simulink model "FlyingSheet_simulator"  (R2019b)
settings: Solver=VariableStepAuto  StartTime=0.0  StopTime=30  RelTol=1e-3
values from neighbouring files (symbols this model uses):
  p =     [ds.mat]    (also in vxs.mat)
undefined symbols (not defined in the file or in its folder): quatnormalize
libraries: aerolibutil x24, simulink x14, sharedtransform x6, vrlib x4, sharedutil x3, simulink_extras x2, dspsrcs4 x1, aerolibanim x1, aerolibanimutils x1
(part 2 of 2)

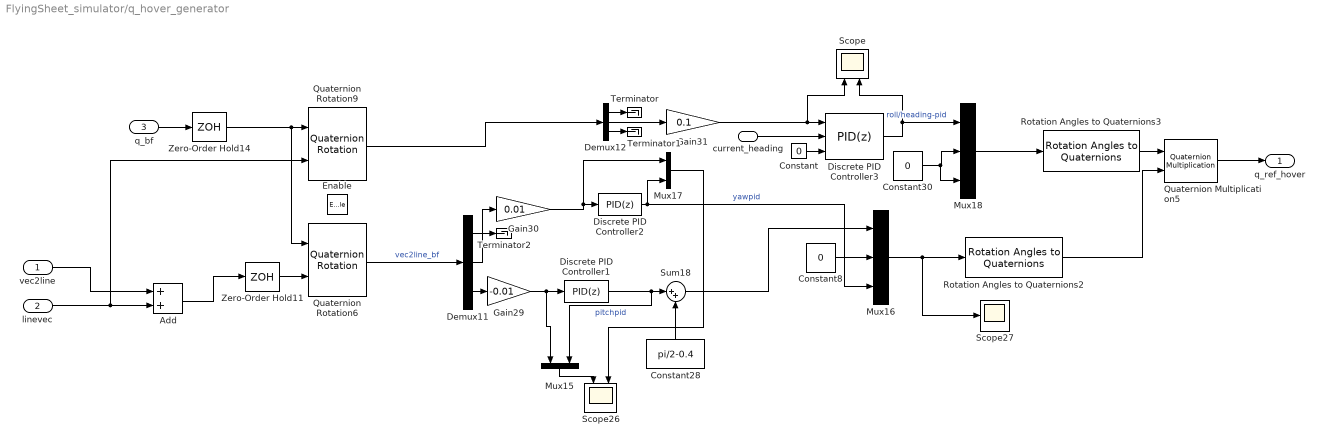
== system FlyingSheet_simulator/q_hover_generator ==
  vec2line : Inport
  linevec : Inport  Port=2
  q_bf : Inport  Port=3
  current_heading : Inport  Port=4
  Enable : EnablePort  StatesWhenEnabling=reset
  Add : Sum
  Constant : Constant  Value=0
  Constant28 : Constant  Value=pi/2-0.4
  Constant30 : Constant  Value=0
  Constant8 : Constant  Value=0
  Demux11 : Demux  Outputs=3
  Demux12 : Demux  Outputs=3
  Discrete PID Controller1 : simulink/Continuous/PID Controller  Controller=PID  Form=Parallel  TimeDomain=Discrete-time  SampleTime=-1  IntegratorMethod=Forward Euler  FilterMethod=Forward Euler  ControllerParametersSource=internal  P=0.75  I=0.1  D=8  UseFilter=off  N=100  TunerSelectOption=Transfer Function Based (PID Tuner App)  InitialConditionSource=internal  InitialConditionForIntegrator=0  InitialConditionForFilter=0  DifferentiatorICPrevScaledInput=0  ExternalReset=none  TrackingMode=off  Kt=1  LimitOutput=on  UpperSaturationLimit=deg2rad(40)  LowerSaturationLimit=-deg2rad(40)  LinearizeAsGain=off  AntiWindupMode=none  Kb=1  POutMin=[]  POutMax=[]  IOutMin=[]  IOutMax=[]  DOutMin=[]  DOutMax=[]  NOutMin=[]  NOutMax=[]  SumOutMin=[]  SumOutMax=[]  SaturationOutMin=[]  SaturationOutMax=[]  PParamMin=[]  PParamMax=[]  IParamMin=[]  IParamMax=[]  DParamMin=[]  DParamMax=[]  NParamMin=[]  NParamMax=[]  KbParamMin=[]  KbParamMax=[]  KtParamMin=[]  KtParamMax=[]  KbOutMin=[]  KbOutMax=[]  KtOutMin=[]  KtOutMax=[]  IntegratorOutMin=[]  IntegratorOutMax=[]  FilterOutMin=[]  FilterOutMax=[]  SumI1OutMin=[]  SumI1OutMax=[]  SumI2OutMin=[]  SumI2OutMax=[]  SumI3OutMin=[]  SumI3OutMax=[]  SumI4OutMin=[]  SumI4OutMax=[]  SumDOutMin=[]  SumDOutMax=[]  DifferentiatorOutMin=[]  DifferentiatorOutMax=[]  FilterDiffOutCoefMin=[]  FilterDiffOutCoefMax=[]  ReciprocalOutMin=[]  ReciprocalOutMax=[]  SumDenOutMin=[]  SumDenOutMax=[]  SumNumOutMin=[]  SumNumOutMax=[]  DivideOutMin=[]  DivideOutMax=[]  IntegratorContinuousStateAttributes=''  IntegratorStateMustResolveToSignalObject=off  IntegratorRTWStateStorageClass=Auto  FilterContinuousStateAttributes=''  FilterStateMustResolveToSignalObject=off  FilterRTWStateStorageClass=Auto  ParallelPVariant=InternalParameters  IdealPVariant=Disabled  IVariant=InternalParameters  DVariant=InternalParameters  IntegratorVariant=Discrete  SatVariant=Enabled  AWVariant=Passthrough  PCopyVariant=Disabled  TRVariant=Disabled  FdbkBlocksVariant=Forward  IdealPFdbkVariant=Disabled  SatFdbkVariant=Disabled  DerivativeFilterVariant=Differentiator  NVariant=Passthrough  NCopyVariant=Disabled_SignalSpec  FilterICVariant=InternalICsDifferentiator  IntegratorICVariant=InternalICs  ExternalResetVariant=Disabled  TRSumVariant=Passthrough  SumFdbkVariant=Disabled  SumVariant=Sum_PID
  Discrete PID Controller2 : simulink/Continuous/PID Controller  Controller=PID  Form=Parallel  TimeDomain=Discrete-time  SampleTime=-1  IntegratorMethod=Forward Euler  FilterMethod=Forward Euler  ControllerParametersSource=internal  P=1  I=0  D=2  UseFilter=off  N=100  TunerSelectOption=Transfer Function Based (PID Tuner App)  InitialConditionSource=internal  InitialConditionForIntegrator=0  InitialConditionForFilter=0  DifferentiatorICPrevScaledInput=0  ExternalReset=none  TrackingMode=off  Kt=1  LimitOutput=on  UpperSaturationLimit=deg2rad(40)  LowerSaturationLimit=-deg2rad(40)  LinearizeAsGain=off  AntiWindupMode=none  Kb=1  POutMin=[]  POutMax=[]  IOutMin=[]  IOutMax=[]  DOutMin=[]  DOutMax=[]  NOutMin=[]  NOutMax=[]  SumOutMin=[]  SumOutMax=[]  SaturationOutMin=[]  SaturationOutMax=[]  PParamMin=[]  PParamMax=[]  IParamMin=[]  IParamMax=[]  DParamMin=[]  DParamMax=[]  NParamMin=[]  NParamMax=[]  KbParamMin=[]  KbParamMax=[]  KtParamMin=[]  KtParamMax=[]  KbOutMin=[]  KbOutMax=[]  KtOutMin=[]  KtOutMax=[]  IntegratorOutMin=[]  IntegratorOutMax=[]  FilterOutMin=[]  FilterOutMax=[]  SumI1OutMin=[]  SumI1OutMax=[]  SumI2OutMin=[]  SumI2OutMax=[]  SumI3OutMin=[]  SumI3OutMax=[]  SumI4OutMin=[]  SumI4OutMax=[]  SumDOutMin=[]  SumDOutMax=[]  DifferentiatorOutMin=[]  DifferentiatorOutMax=[]  FilterDiffOutCoefMin=[]  FilterDiffOutCoefMax=[]  ReciprocalOutMin=[]  ReciprocalOutMax=[]  SumDenOutMin=[]  SumDenOutMax=[]  SumNumOutMin=[]  SumNumOutMax=[]  DivideOutMin=[]  DivideOutMax=[]  IntegratorContinuousStateAttributes=''  IntegratorStateMustResolveToSignalObject=off  IntegratorRTWStateStorageClass=Auto  FilterContinuousStateAttributes=''  FilterStateMustResolveToSignalObject=off  FilterRTWStateStorageClass=Auto  ParallelPVariant=InternalParameters  IdealPVariant=Disabled  IVariant=InternalParameters  DVariant=InternalParameters  IntegratorVariant=Discrete  SatVariant=Enabled  AWVariant=Passthrough  PCopyVariant=Disabled  TRVariant=Disabled  FdbkBlocksVariant=Forward  IdealPFdbkVariant=Disabled  SatFdbkVariant=Disabled  DerivativeFilterVariant=Differentiator  NVariant=Passthrough  NCopyVariant=Disabled_SignalSpec  FilterICVariant=InternalICsDifferentiator  IntegratorICVariant=InternalICs  ExternalResetVariant=Disabled  TRSumVariant=Passthrough  SumFdbkVariant=Disabled  SumVariant=Sum_PID
  Discrete PID Controller3 : simulink/Continuous/PID Controller  Controller=PID  Form=Parallel  TimeDomain=Discrete-time  SampleTime=-1  IntegratorMethod=Forward Euler  FilterMethod=Forward Euler  ControllerParametersSource=internal  P=1  I=1  D=0  UseFilter=off  N=100  TunerSelectOption=Transfer Function Based (PID Tuner App)  InitialConditionSource=external  InitialConditionForIntegrator=0  InitialConditionForFilter=0  DifferentiatorICPrevScaledInput=0  ExternalReset=none  TrackingMode=off  Kt=1  LimitOutput=off  UpperSaturationLimit=deg2rad(40)  LowerSaturationLimit=-deg2rad(40)  LinearizeAsGain=off  AntiWindupMode=none  Kb=1  POutMin=[]  POutMax=[]  IOutMin=[]  IOutMax=[]  DOutMin=[]  DOutMax=[]  NOutMin=[]  NOutMax=[]  SumOutMin=[]  SumOutMax=[]  SaturationOutMin=[]  SaturationOutMax=[]  PParamMin=[]  PParamMax=[]  IParamMin=[]  IParamMax=[]  DParamMin=[]  DParamMax=[]  NParamMin=[]  NParamMax=[]  KbParamMin=[]  KbParamMax=[]  KtParamMin=[]  KtParamMax=[]  KbOutMin=[]  KbOutMax=[]  KtOutMin=[]  KtOutMax=[]  IntegratorOutMin=[]  IntegratorOutMax=[]  FilterOutMin=[]  FilterOutMax=[]  SumI1OutMin=[]  SumI1OutMax=[]  SumI2OutMin=[]  SumI2OutMax=[]  SumI3OutMin=[]  SumI3OutMax=[]  SumI4OutMin=[]  SumI4OutMax=[]  SumDOutMin=[]  SumDOutMax=[]  DifferentiatorOutMin=[]  DifferentiatorOutMax=[]  FilterDiffOutCoefMin=[]  FilterDiffOutCoefMax=[]  ReciprocalOutMin=[]  ReciprocalOutMax=[]  SumDenOutMin=[]  SumDenOutMax=[]  SumNumOutMin=[]  SumNumOutMax=[]  DivideOutMin=[]  DivideOutMax=[]  IntegratorContinuousStateAttributes=''  IntegratorStateMustResolveToSignalObject=off  IntegratorRTWStateStorageClass=Auto  FilterContinuousStateAttributes=''  FilterStateMustResolveToSignalObject=off  FilterRTWStateStorageClass=Auto  ParallelPVariant=InternalParameters  IdealPVariant=Disabled  IVariant=InternalParameters  DVariant=InternalParameters  IntegratorVariant=Discrete  SatVariant=Disabled  AWVariant=Passthrough  PCopyVariant=Disabled  TRVariant=Disabled  FdbkBlocksVariant=Forward  IdealPFdbkVariant=Disabled  SatFdbkVariant=Disabled  DerivativeFilterVariant=Differentiator  NVariant=Passthrough  NCopyVariant=Disabled_SignalSpec  FilterICVariant=ExternalICs  IntegratorICVariant=ExternalICs  ExternalResetVariant=Disabled  TRSumVariant=Passthrough  SumFdbkVariant=Disabled  SumVariant=Sum_PID
  Gain29 : Gain  Gain=-0.01
  Gain30 : Gain  Gain=0.01
  Gain31 : Gain  Gain=0.1
  Mux15 : Mux  Inputs=2
  Mux16 : Mux  Inputs=3
  Mux17 : Mux  Inputs=2
  Mux18 : Mux  Inputs=3
  Quaternion Multiplication5 : aerolibutil/Quaternion Multiplication
  Quaternion Rotation6 : aerolibutil/Quaternion Rotation
  Quaternion Rotation9 : aerolibutil/Quaternion Rotation
  Rotation Angles to Quaternions2 : sharedtransform/Rotation Angles to Quaternions  rotationOrder=YXZ  aMode=aMode
      settings: SourceProductName=Aerospace Blockset  SourceProductBaseCode=AE
  Rotation Angles to Quaternions3 : sharedtransform/Rotation Angles to Quaternions  rotationOrder=ZYX  aMode=aMode
      settings: SourceProductName=Aerospace Blockset  SourceProductBaseCode=AE
  Scope : Scope  NumInputPorts=2
  Scope26 : Scope  NumInputPorts=2
  Scope27 : Scope
  Sum18 : Sum  Inputs=|++
  Terminator : Terminator
  Terminator1 : Terminator
  Terminator2 : Terminator
  Zero-Order Hold11 : ZeroOrderHold  SampleTime=p.Ts
  Zero-Order Hold14 : ZeroOrderHold  SampleTime=p.Ts
  q_ref_hover : Outport  VectorParamsAs1DForOutWhenUnconnected=off
  wires:
  vec2line/1 -> Add/1
  Discrete PID Controller1/1 -> Sum18/1, Mux15/2  "pitchpid"
  Gain29/1 -> Mux15/1, Discrete PID Controller1/1
  Demux11/2 -> Gain30/1
  Quaternion Rotation6/1 -> Demux11/1  "vec2line_bf"
  Constant30/1 -> Mux18/3, Mux18/2
  Demux12/3 -> Terminator1/1
  Demux12/1 -> Terminator/1
  Gain31/1 -> Scope/1, Discrete PID Controller3/1
  linevec/1 -> Quaternion Rotation9/2, Add/2
  Discrete PID Controller3/1 -> Scope/2, Mux18/1  "roll/heading-pid"
  Mux15/1 -> Scope26/1
  Mux16/1 -> Scope27/1, Rotation Angles to Quaternions2/1
  Rotation Angles to Quaternions3/1 -> Quaternion Multiplication5/1
  q_bf/1 -> Zero-Order Hold14/1
  Demux11/3 -> Gain29/1
  Constant8/1 -> Mux16/2
  Discrete PID Controller2/1 -> Mux16/3, Mux17/2  "yawpid"
  Rotation Angles to Quaternions2/1 -> Quaternion Multiplication5/2
  Mux18/1 -> Rotation Angles to Quaternions3/1
  Quaternion Multiplication5/1 -> q_ref_hover/1
  Demux12/2 -> Gain31/1
  Mux17/1 -> Scope26/2
  Add/1 -> Zero-Order Hold11/1
  Zero-Order Hold14/1 -> Quaternion Rotation6/1, Quaternion Rotation9/1
  Constant28/1 -> Sum18/2
  Gain30/1 -> Mux17/1, Discrete PID Controller2/1
  Zero-Order Hold11/1 -> Quaternion Rotation6/2
  Demux11/1 -> Terminator2/1
  Sum18/1 -> Mux16/1
  Constant/1 -> Discrete PID Controller3/3
  current_heading/1 -> Discrete PID Controller3/2
  Quaternion Rotation9/1 -> Demux12/1

== matlab function FlyingSheet_simulator/Torque_FL ==
  data: u_omegaL output; u_omegaR output; u_deltaL output; u_deltaR output; tao input; states input; u_jointT input; p parameter
function [u_omegaL,u_omegaR, u_deltaL,u_deltaR]  = FL_torques(tao, states, u_jointT, p)


wxr = tao(1); % I wonder if this comversion from omega to tao is right? Depends on Emil Fresk implementation
wyr = tao(2);
wzr = tao(3);
v = states(1:3);
vx = v(1);
vy = v(2);
vz = v(3);
w = states(4:6);
wx = w(1);
wy = w(2);
wz = w(3);
q = states(7:10); % Possibly not needed?
q0=q(1);
q1=q(2);
q2=q(3);
q3=(4);
deltaL = states(11);
deltaR = states(12);
omegaL = states(13);
omegaR = states(14);

% init output vector
u_deltaL = 0;
u_deltaR = 0;
u_omegaL = 0;
u_omegaR = 0;

% If you know of a better way (not counting modifying the code below to use
% p.x notation, plese feel welcome to tell me.
%P = struct2cell(p);
%Pn = fieldnames(p);
%for i=1:numel(P)
%    eval(Pn{i}+"="+string(P{i})+";")
%end
Ts=p.Ts;
m=p.m;
Ix=p.Ix;
Iy=p.Iy;
Iz=p.Iz;
I=p.I;
g=p.g;
rho=p.rho;
propd=p.propd;
K_T=p.K_T;
K_v=p.K_v;
b_w=p.b_w;
Sa=p.Sa;
Saw=p.Saw;
CLdelta=p.CLdelta;
CDdelta=p.CDdelta;
SW=p.SW;
Sw_w=p.Sw_w;
Sw=p.Sw;
b=p.b;
Cmyl=p.Cmyl;
Cwy=p.Cwy;
yf=p.yf;
yt=p.yt;
xW=p.xW;
xf=p.xf;
xac=p.xac;
zW=p.zW;
yw=p.yw;
yW=p.yW;
yWE=p.yWE;
yWEE=p.yWEE;
K_omegaL=p.K_omegaL;
K_omegaR=p.K_omegaR;
K_deltaL=p.K_deltaL;
K_deltaR=p.K_deltaR;
CL_A=p.CL_A;
CL_B=p.CL_B;
CL_C=p.CL_C;
CD_A=p.CD_A;
CD_B=p.CD_B;
CD_C=p.CD_C;
CLB_A=p.CLB_A;
CLB_B=p.CLB_B;
CDB_A=p.CDB_A;
CDB_B=p.CDB_B;
% The constants below are for the polynomial approximations.
% I am lookin into a way of auto-generating them in a struct or something.
a11=p.a11;
a12=p.a12;
a13=p.a13;
a21=p.a21;
a22=p.a22;
a23=p.a23;
a31=p.a31;
a32=p.a32;
a33=p.a33;
a41=p.a41;
a42=p.a42;
a43=p.a43;
b11=p.b11;
b12=p.b12;
b13=p.b13;
b14=p.b14;
b21=p.b21;
b22=p.b22;
b23=p.b23;
b24=p.b24;
b31=p.b31;
b32=p.b32;
b33=p.b33;
b34=p.b34;
c11=p.c11;
c12=p.c12;
c13=p.c13;
c14=p.c14;
c21=p.c21;
c22=p.c22;
c23=p.c23;
c24=p.c24;
c31=p.c31;
c32=p.c32;
c33=p.c33;
c34=p.c34;
c41=p.c41;
c42=p.c42;
c43=p.c43;
c44=p.c44;
% Assuming we made correct choices here it should suffice with this:
%u = [u_deltaA u_jointA u_deltaT]';


% Hey, anyone reading this? Code below is auto-generated because the
% F.L. was just too much of a headache to do
% manyally, so I wrote a script for it.
wn = p.wn;
u_ref =[ ...
];
 
u_deltaA = u_ref(1);
u_jointA = u_ref(2);
u_deltaT = u_ref(3);

u_deltaL = u_jointA - u_deltaA/2;
u_deltaR = u_jointA + u_deltaA/2;
u_omegaL = u_jointT + u_deltaT/2;
u_omegaR = u_jointT - u_deltaT/2;

gain = 1;
u_deltaL = gain*u_deltaL;
u_deltaR = gain*u_deltaR;

end

== matlab function FlyingSheet_simulator/TailSitter/tailsittersimv2 ==
  data: omegaLdot output; omegaRdot output; deltaLdot output; deltaRdot output; qdot output; wdot output; vdot output; omegaL input; omegaR input; deltaL input; deltaR input; u_omegaL input; u_omegaR input; u_deltaL input; u_deltaR input; q input; w input; v input; wind_v input; p parameter; alpha output; Beta output; g_out output
function [ omegaLdot, omegaRdot, deltaLdot, deltaRdot, qdot,wdot,vdot, alpha, Beta, g_out] = ...
    tailsitter_v2(omegaL, omegaR, deltaL, deltaR, u_omegaL, u_omegaR, u_deltaL, ...
    u_deltaR, q,w,v, wind_v, p)

% Set output port dim
omegaLdot = 0;
omegaRdot = 0;
deltaLdot = 0;
deltaRdot = 0;
alpha = 0;
Beta = 0;
qdot = zeros(4,1);
wdot = zeros(3,1);
vdot = zeros(3,1);
g_out = zeros(3,1);

% Map inputs
vx = v(1) + wind_v(1);
vy = v(2) + wind_v(2);
vz = v(3) + wind_v(3);

wx = w(1);
wy = w(2);
wz = w(3);

q0 = q(1);
q1 = q(2);
q2 = q(3);
q3 = q(4);

% function handles not supported, so adding here directly
c = @(y) 0.39; % This should be pretty accurate
% Lift curves
CL = @(alpha) p.CL_A*sin(p.CL_B.*alpha)+p.CL_C; % These are wrong, just placeholders
CD = @(alpha) p.CD_A-p.CD_A.*cos(p.CD_B.*alpha)+p.CD_C;

alpha = atan2(vz,vx);

%Thrust
TL = p.K_T .* omegaL.^2;
TR = p.K_T .* omegaR.^2;

% airflow in thrust wake
v_w_L = p.b_w .* omegaL; %[b_w .* omegaL; vy; vz];
v_w_R = p.b_w .* omegaR;
%alpha_wL = atan2(vz,v_w_L);
%alpha_wR = atan2(vz,v_w_R);

% Quaternion
qdot = 0.5.*[-q1 -q2 -q3; ...
            q0 -q3 q2; ...
            q3 q0 -q1; ...
            -q2 q1 q0]*w;

% inputs
deltaLdot = p.K_deltaL .* (-deltaL + u_deltaL);
deltaRdot = p.K_deltaR .* (-deltaR + u_deltaR);
omegaLdot = p.K_omegaL .* (-omegaL + u_omegaL);
omegaRdot = p.K_omegaR .* (-omegaR + u_omegaR);

% gravity
% To get vector g in bf from wf
% we need to rotate it by q_wf, or conj(q_bf)
qc = quatconj([q0 q1 q2 q3]); %
qc0 = qc(1);
qc1 = qc(2);
qc2 = qc(3);
qc3 = qc(4);
gravity = p.g .* [2.*(qc1.*qc3 + qc0.*qc2); ...
                2.*(qc2.*qc3 - qc0.*qc1); ...
                (qc0.^2 - qc1.^2 - qc2.^2 + qc3.^2);
                zeros(3+4+4,1)];
g_out = gravity(1:3,1);
% Inertial forces
inertialF = -[2*(vz.*wy - vy.*wz); ...
             2*(vx.*wz - vz.*wx); ...
             2*(vy.*wx - vx.*wy); ...
             (p.Iz - p.Iy).*wy.*wz./p.Ix; ...
             (p.Ix - p.Iz).*wx.*wz./p.Iy; ...
             (p.Iy - p.Ix).*wx.*wy./p.Iz; ...
             zeros(8,1)];
%Sideslip
Beta = atan2(vy,vx);

% Winglets
CLB = @(beta) p.CLB_A*sin(p.CLB_B.*beta); % These are wrong, just placeholders
CDB = @(beta) p.CDB_A-p.CDB_A.*cos(p.CDB_B.*beta);
L_W = -p.rho * sqrt(vx.^2+vy.^2) * p.SW * (CLB(Beta)*vx + CDB(Beta)*vy); % Lift in bodyframe, y
D_W = p.rho * sqrt(vx.^2+vy.^2) * p.SW * (-CLB(Beta)*vy + CDB(Beta)*vx); % Drag in bodyfram, x

% MAIN WING
% Lift inside wake
LLT = p.Sw_w * 0.5 * p.rho * abs(v_w_L) .* CL(0).*v_w_L ;
LRT = p.Sw_w * 0.5 * p.rho * abs(v_w_R) .* CL(0).*v_w_R ;
% Lift outside wake
LL = p.Sw * 0.5 * p.rho * sqrt(vx.^2 + vz.^2) .* ...
    (CL(alpha).*vx + CD(alpha).*vz);
LR = LL; % Yeah we -could- combine these, but too late!
% Drag inside wake
DLT = p.Sw_w * 0.5 * p.rho * abs(v_w_L) * CD(0) * v_w_L;
DRT = p.Sw_w * 0.5 * p.rho * abs(v_w_R) * CD(0) * v_w_R;
% Drag outside wake
DL = p.Sw * 0.5 * p.rho * sqrt(vx.^2  + vz.^2) .* ...
    (-CL(alpha).*vz + CD(alpha).*vx);
DR = DL; % Yeah, we -could- combine these as well...

% AILERONS
% Lift inside wake, signs bc rotation dir of aileron
FLT = -p.CLdelta * 0.5*p.rho*v_w_L.^2 * p.Saw * deltaL;
FRT = -p.CLdelta * 0.5*p.rho*v_w_R.^2 * p.Saw * deltaR;
% Lift outside wake
FL = -sign(vx).*p.CLdelta * 0.5*p.rho*(vx.^2 + vy.^2 + vz.^2) * p.Sa * deltaL;
FR = -sign(vx).*p.CLdelta * 0.5*p.rho*(vx.^2 + vy.^2 + vz.^2) * p.Sa * deltaR;
% Drag inside wake
DalphaLT =p.CDdelta * 0.5*p.rho*v_w_L.^2 * p.Saw * abs(deltaL);
DalphaRT = p.CDdelta * 0.5*p.rho*v_w_R.^2 * p.Saw * abs(deltaR);
% Drag outside wake, we add sign of vx because we might be reversing?
DalphaL = sign(vx).*p.CDdelta * 0.5*p.rho*(vx.^2 + vy.^2 + vz.^2) * p.Sa * abs(deltaL);
DalphaR = sign(vx).*p.CDdelta * 0.5*p.rho*(vx.^2 + vy.^2 + vz.^2) * p.Sa * abs(deltaR);

% f1
 % diff in ail deflection
  % inside wake
  % outside wake
 % resmom roll,
 % roll due to yaw rate
 % moment due to sideslip
alphal_rmr = @(y) atan2(vz+wx.*y, vx);
restmomroll = @(y) y .* c(y) .* sqrt(vx.^2 + (vz+wx.*y).^2) .* ...
    (CL(alphal_rmr(y)).*vx + CD(alphal_rmr(y)).*(vz+wx.*y));
alphal_rwz = @(y) atan2(vz, vx-wz.*y);
rollduetowz = @(y) y .* c(y) .* sqrt((vx-wz.*y).^2 + vz.^2) .* ...
    (CL(alphal_rwz(y)).*(vx-wz*y) + CD(alphal_rwz(y)).*vz);
f1 = p.yf.*(FLT+FL -FRT-FR) ...
    -0.5*p.rho.*quadgk(restmomroll,-p.yW,p.yW) ... % between wakes
     -0.5*p.rho.*quadgk(restmomroll,-p.yWEE,-p.yWE) ... % outside left wake
      -0.5*p.rho.*quadgk(restmomroll,p.yWE,p.yWEE) ... % outside right wake
    -0.5*p.rho.*quadgk(rollduetowz,-p.yW,p.yW) ... between wakes
     -0.5*p.rho.*quadgk(rollduetowz,-p.yWEE,-p.yWE) ... left side
      -0.5*p.rho.*quadgk(rollduetowz, p.yWE,p.yWEE) ... right side
    +p.zW*L_W;
% f2
 % joint ail deflection
  % inside wake
  % outside wake
 % pitch moment
 % restmom pitch rate, --- compensate for wake!
 % Pitch from winglets
f2 = p.xf.*(FLT+FL+FRT+FR) ...
    ... %+ 0.5*p.rho*p.Cmyl*(2*p.Sw.*(vx.^2+vy.^2+vz.^2)+p.Sw_w*(v_w_L.^2 + v_w_R.^2) ) ...
    -p.xac.*(LL+LR+LLT+LRT) ... % We do not assume Pith coeff static.
    -wy.*p.rho.*2.*p.Sw.*p.Cwy.*sqrt(vx.^2 + vz.^2) ...
    +p.zW*D_W;
% f3
 % diff in T
 % mom due to sideslip
 % restmom yaw rate, compensate for outside wake
restmomwz = @(y) y .* c(y) .* sqrt((vx-wz.*y).^2 + vz.^2) .* ...
    (-CL(alphal_rwz(y)).*vz + CD(alphal_rwz(y)).*(vx-wz.*y));
f3 = p.yt.*(TL-TR) ...
     -p.xW*L_W ...
     +0.5*quadgk(restmomwz,-p.yW,p.yW) ...
     +0.5*quadgk(restmomwz,-p.yWEE,-p.yWE) ...
     +0.5*quadgk(restmomwz, p.yWE,p.yWEE);
 
%velocities
vxdot = (TL +TR -DL -DR -DLT -DRT -D_W -DalphaL -DalphaR -DalphaLT -DalphaRT)./p.m;
vydot = L_W./p.m;
vzdot = (-LL -LR -LLT -LRT +FL +FR +FLT +FRT)./p.m;

% angular rates
wxdot = f1./p.Ix;
wydot = f2./p.Iy;
wzdot = f3./p.Iz;

%if any(abs(vxdot) > 100)
%    p.m
%end

statesdot = gravity + inertialF +  ...
    [vxdot;vydot;vzdot;wxdot;wydot;wzdot;qdot;...
    deltaLdot;deltaRdot;omegaLdot;omegaRdot];

vdot = statesdot(1:3);
wdot = statesdot(4:6);
qdot = statesdot(7:10);
deltaLdot = statesdot(11);
deltaRdot = statesdot(12);
omegaLdot = statesdot(13);
omegaRdot = statesdot(14);

== matlab function FlyingSheet_simulator/TailSitter/myQuatNorm ==
  data: q input; n output
function n = fcn(q)

n = sqrt(q(1).^2 + q(2).^2 + q(3).^2 + q(4).^2);

== matlab function FlyingSheet_simulator/MATLAB Function ==
  data: u input; y output
function y = norm(u)

y = sqrt(sum(u.^2));

== matlab function FlyingSheet_simulator/TailSitter/MATLAB Function ==
  data: time input; w output
function w = rotsteps(time)

stept = 10;
wt = 10;
reverse = 0;
if time<stept
    w = [0.1,0,0];
elseif time<stept+wt
    if reverse
        w = [-0.1,0,0];
    else
        w = zeros(1,3);
    end
elseif time<2*stept+wt
    w = [0,0,0.1];
elseif time<2*stept+2*wt
    if reverse
        w = [0,0,-0.1];
    else
        w = zeros(1,3);
    end
else
    w = [0,0.1,0];
end

== matlab function FlyingSheet_simulator/MATLAB Function2 ==
  data: q_wf input; q_ref output
function q_ref = refquat(q_wf)

% TODO: Figure out how to set a good reference quaternion.
q_ref = q_wf;

== matlab function FlyingSheet_simulator/MATLAB Function1 ==
  data: v_ref input; q_ref output; u_jointT output
function [q_ref,u_jointT] = ref_quat(v_ref)


q_ref = [1,0,0,0]';
u_jointT = 300;

% We have output of 5dof.
% Input is 3dof.
% We can extend input dof by saying we want wings to be horizontal, now
% total in is 4dof.


%Construct quaterion from several different rotations?

== matlab function FlyingSheet_simulator/linegenerator ==
  settings: updateMethod=DISCRETE
  data: v_wf input; r input; p parameter; rspeed output; wpN output; dist2wp output; linevec output; vec2line output; wp_r output
function [rspeed,wpN, dist2wp, linevec, vec2line, wp_r] = LineGenerator( v_wf,r, p)

% Keep track of which waypoint we are going to
persistent waypointno;
persistent wp;
persistent wp_prev;
persistent miss;
if isempty(waypointno)
    waypointno=2;
    wp=p.waypoints(waypointno,:)';
    wp_prev=p.waypoints(waypointno-1,:)';
    miss=0;
end

%initialize variables
dist2line2d = 0;
altError = 0;
thetaerr = 0;
rspeed = 0;
vec2line = [0,0,0]';

% if current waypoint is the start wp/home wp jump immediately to next.
dist2wp = sqrt( sum( (wp(1:3)-r).^2 ) );
if dist2wp <= wp(5)
    if waypointno < p.numwp
        waypointno = waypointno+1;
    else
        waypointno = 2; % we always skip home wp at origin
    end
    wp_prev = wp;
    wp = p.waypoints(waypointno,:)';
    miss=0;
end
rspeed = wp(4);
wp_r = wp(1:3); % Next waypoint position, v has been scaled away thus wp_r

% find vector between last waypoint and current target
linevec = (wp(1:3)-wp_prev(1:3))./sqrt( sum((wp(1:3)-wp_prev(1:3)).^2) );

% Check if we missed our goal!
%{
if ~miss && dot(linevec, wp(1:3)-r) < 0 && sqrt(sum( (wp(1:3)-r).^2 )) > wp(5)*2
    linevec(1:2)=-linevec(1:2);
    miss=1;
elseif miss
    linevec(1:2)=-linevec(1:2);
end
%}
if  dot(linevec, wp(1:3)-r) < 0 
    linevec(1:3)=-linevec(1:3);
end
% Figure out if goal is ahead of us or if we passed it/missed it.
%if dot(v_wf(1:3), wp(1:3)-r(1:3)) < 0
%    linevec(1:2) = - linevec(1:2);
%end
% THe above doesn't work.

%{
% find angle in x-y plane of vector
thetastar = atan2(linevec(2), linevec(1));
% find our current heading
theta = atan2(v_wf(2),v_wf(1));
% Error in direction along line / be paralell with line
thetaerr = thetastar - theta;
%}

% Find the vector that describes the vector to the closest point on the
% line
a = wp_prev(1:3);               % Points to "start of line"
n = linevec;                    % Points toward next wp
vec2line = a-r - dot(a-r,n)*n;
%altError = vec2line(3);
%dist2line2d = sqrt( sum( vec2line(1:2).^2 ));
wpN = waypointno;


% Mix the vectors for reference according to how far away from line we are

% Old setup, constants: 0.0075/0.01, max/dl2coeff
%{
%cr = cross(linevec,vec2line);
%refvec = linevec;
vcomp = (12/rspeed).^2;
if abs(d2lcoeff*dist2line2d) < max2l*vcomp
    refvec = linevec + d2lcoeff*dist2line2d*vec2line;
else
    refvec = linevec + vcomp*max2l*vec2line;
end
}
%}

%{
vcomp=1/rspeed;
refvec = linevec+vec2line*d2lcoeff*vcomp;

refvec = refvec/sqrt(sum(refvec.^2));
%}

== matlab function FlyingSheet_simulator/q_fly_generator/MATLAB Function3 ==
  data: pitchPID input; vherror output; pitch output; vr_wf input; v_wf input
function [vherror,pitch] = setpitch(pitchPID,vr_wf, v_wf)

pitch = 0;

% Angle toward horizon given by:
horzspeedr = sqrt(sum(vr_wf(1:2).^2));  % Horizontal speed requested
pitch = (horzspeedr +6.013)/15.38;      % From simulations and linefitting
pitch = (pi/2-pitch);                   % correct for coordsys

% We can choose:
%   - Regulate horizontal speed with pitch and altitude with engine power
%   - Regulate horizontal speed with engine power and altitude with pitch.
%
% The first option makes sense when hovering but may be problematic when
% flying: if we are horizontally oriented and dropping in altitude engine
% power cannot do anything about it. However, it will try to increase speed
% forcing the pitch controller to pitch up to reduce speed. Might work.
% The second option makes sense when flying. When hovering we have no
% horizontal speed though.
%

horzspeed  = sqrt(sum( v_wf(1:2).^2));  % Actual horizontal speed
vherror = horzspeedr-horzspeed;         % Error in horizontal speed, to be
                                        % sent to externa PID.

% correct pitch using measurments, use external pid
pitch = pitch + pitchPID;


% use error in direction to roll slightly, use external PID
%roll = 0.1*yawe;

== matlab function FlyingSheet_simulator/MATLAB Function9 ==
  data: q_fly input; vr_wf input; v_cutoff input; q_ref output; q_hover input; hovermode output
function [q_ref, hovermode] = modeswitcher(q_fly, vr_wf, v_cutoff, q_hover)

hspeed = sqrt(sum( vr_wf(1:2).^2 ));
vspeed = abs(vr_wf(3));

Theta = atan2(hspeed, vspeed);

rspeed = sqrt(sum( vr_wf.^2 ));
if rspeed < v_cutoff || abs(Theta) < deg2rad(20)
    q_ref = q_hover;
    hovermode = 1;
else
    q_ref = q_fly;
    hovermode=0;
end

== matlab function FlyingSheet_simulator/linegenerator1 ==
  settings: updateMethod=DISCRETE
  data: max2l input; d2lcoeff input; r input; altError output; p parameter; rspeed output; refvec output; wpN output; dist2wp output; vec2line output
function [altError, rspeed, refvec, wpN, dist2wp, vec2line] = LineGenerator(max2l, d2lcoeff ,r,p)

% Keep track of which waypoint we are going to
persistent waypointno;
persistent wp;
persistent wp_prev;
if isempty(waypointno)
    waypointno = 1;
    wp = p.waypoints(waypointno,:)';
    wp_prev = p.waypoints(waypointno,:)';
end

%initialize variables
dist2line2d = 0;
altError = 0;
rspeed = 0;
vec2line = [0,0,0]';

% if current waypoint is the start wp/home wp jump immediately to next.
dist2wp = sqrt( sum( (wp(1:3)-r).^2 ) );
if dist2wp <= p.wpradius
    if waypointno < p.numwp
        waypointno = waypointno+1;
    else
        waypointno = 1; 
    end
    wp_prev = wp;
    wp = p.waypoints(waypointno,:)';
end
rspeed = wp(4);

% find vector between last waypoint and current target
linevec = (wp(1:3)-wp_prev(1:3))./sqrt( sum((wp(1:3)-wp_prev(1:3)).^2) );

% Figure out if goal is ahead of us or if we passed it/missed it.
%if dot(v_wf(1:3), wp(1:3)-r(1:3)) < 0
%    linevec(1:2) = - linevec(1:2);
%end
% THe above doesn't work.


% Find the vector that describes the vector to the closest point on the
% line
a = wp_prev(1:3);
n = linevec;
vec2line = a-r - dot(a-r,n)*n;
altError = vec2line(3);
dist2line2d = sqrt( sum( vec2line(1:2).^2 ));
wpN = waypointno;


% Mix the vectors for reference according to how far away from line we are
%cr = cross(linevec,vec2line);
%refvec = linevec;
if abs(d2lcoeff*dist2line2d) < max2l
    refvec = linevec + d2lcoeff*dist2line2d*vec2line;
else
    refvec = linevec + max2l*vec2line;
end
refvec = refvec/sqrt(sum(refvec.^2));

== matlab function FlyingSheet_simulator/q_fly_generator/ZYX-quat ==
  data: y input; z input; q output; x input
function q = rotang2quat(y,z,x)

q = [0,0,0,0];

u = [z,y,x];
qa = quaternion(u, 'euler', 'ZYX', 'frame');
q = qa.compact;

== matlab function FlyingSheet_simulator/q_fly_generator/MATLAB Function5 ==
  data: yawr input; yaw input; yawe output
function yawe = fcn(yawr,yaw)

% IF our angle error is more than 180 degrees we need to cross the sign
% barrier, this code should take care of that.
% Since rate limiters are in play, we might need to loo at yawr_target, but
% lets wait with that for now.

yawe = yawr-yaw;
% r:100, y:-90 => e=190 => -360+190= -170
% r:-100, y=90 => e=-190 => 360+(-190) = 170
if yawe > pi
    yawe = -2*pi+yawe;
elseif yawe < -pi
    yawe = 2*pi+yawe;
end

== matlab function FlyingSheet_simulator/q_fly_generator/MATLAB Function6 ==
  data: yawr input; maxrate input; yawr_last input; yawr_slow output; p parameter
function yawr_slow  = fcn(yawr, maxrate, yawr_last, p)

%This is a rate limiter that takes into account which direction is closest
%to the reference, i.e. makes sure we cross the sign at +-pi if we need to.

% We would like to set yawr_slow to yawr, but can only approach it in steps
% of maxrate.
yawr_slow = yawr;
e = yawr-yawr_last;
% slew rate = unit/s => (unit*sampletime)/s
maxrate = maxrate*p.Ts;

if abs(e) > maxrate
    if e > pi
        yawr_slow = yawr_last - maxrate;
    elseif e < -pi
        yawr_slow = yawr_last + maxrate;
    else
        yawr_slow = yawr_last + sign(e)*maxrate;
    end
end

while(yawr_slow > pi)
    yawr_slow = yawr_slow - 2*pi;
end
while(yawr_slow < -pi)
    yawr_slow = yawr_slow + 2*pi;
end

end

== matlab function FlyingSheet_simulator/MATLAB Function7 ==
  data: refvec input; qref output
function qref = refvec2refquat(refvec)

qref = [0,0,0,0];

% set yaw correct
if sqrt(sum( refvec(1:2).^2 )) < 0.1 % Check if we are only pointing up
    Y = 0;
else
    Y = atan2(refvec(2),refvec(1));
end
qY = [cos(Y/2),0,0,sin(Y/2)];

% set pitch correct
hspeed = sqrt(sum(refvec(1:2)).^2);
T = atan2(refvec(3),hspeed);
qT = [cos(T/2),0,sin(T/2),0];


% Set roll to horizontal
qR = [1,0,0,0];

qref = quatmultiply(quatmultiply(qY,qT), qR);

== matlab function FlyingSheet_simulator/q_fly_generator/MATLAB Function8 ==
  data: vr_wf input; yawr output; v_wf input; yaw output
function [yawr,yaw] = setyaw(vr_wf,v_wf)

% reference heading
yawr = atan2(vr_wf(2),vr_wf(1));
%current heading
 yaw = atan2(v_wf(2),v_wf(1));

== matlab function FlyingSheet_simulator/FlyVecAdjust ==
  data: rspeed input; refvec output; vec2line input; linevec input; d2lcoeff input
function refvec = flyVecAdjust(rspeed, vec2line,linevec, d2lcoeff)

vcomp=1/rspeed;
refvec = linevec+vec2line*d2lcoeff*vcomp;

refvec = refvec/sqrt(sum(refvec.^2));

== matlab function FlyingSheet_simulator/MATLAB Function11 ==
  data: P input; D input; axisgains input; angErr input; taos output; w input
function taos = taos_fordecoupler(P, D, axisgains,angErr, w)

taos = [0;0;0];

P1 = P; %4; %30;
P2 = D; %0.3; %=4*3*1/40; %7.5;
cx = axisgains(1);%10;
cy = axisgains(2);%100;
cz = axisgains(3);%1;


% Emil Fresk P2 controller
taos = -P1.*angErr - P2.*w;
% Adjustment for actuators
taos(1) = cx*taos(1);
taos(2) = cy*taos(2);
taos(3) = cz*taos(3);

== matlab function FlyingSheet_simulator/MATLAB Function12 ==
  data: hovermode input; c output; c_hov input; max_hov input; c_fly input; max_fly input; max output
function [c, max] = fcn(hovermode, c_hov, max_hov, c_fly, max_fly)

if hovermode
    c = c_hov;
    max = max_hov;
else
    c = c_fly;
    max = max_fly;
end

== matlab function FlyingSheet_simulator/AdHoc2 ==
  data: u_jointT input; u_omegaL output; u_omegaR output; u_deltaL output; u_deltaR output; tx input; ty input; tz input
function [u_omegaL,u_omegaR, u_deltaL,u_deltaR]  = AdHocTorques( u_jointT, tx, ty, tz)

% This is a crude/simple input/output/actuator linker.
% A pitch torque is made by moving elevons in the same direction: jointA.
% A roll torque is made by moving elevons in opposite direction: deltaA.
% A yaw torque is made by a differential thrust of the engines: deltaT.
% Power forward is given and passed straight through this function as
% jointT.

u_deltaL = 0;
u_deltaR = 0;
u_omegaL = 0;
u_omegaR = 0;



u_deltaA = -tx;
u_jointA = -ty;
u_deltaT = -tz;

u_deltaL = u_jointA - u_deltaA/2;
u_deltaR = u_jointA + u_deltaA/2;
u_omegaL = u_jointT + u_deltaT/2;
u_omegaR = u_jointT - u_deltaT/2;


end

== matlab function FlyingSheet_simulator/MATLAB Function3 ==
  data: v_wf input; yaw output; vr_wf input
function yaw = fcn(v_wf, vr_wf)

yawr = atan2(vr_wf(2),vr_wf(1));

if abs(atan2(sqrt(sum(v_wf(1:2).^2)),abs(v_wf(3)))) < 0.1
    yaw = yawr;
else
    yaw = atan2(v_wf(2),v_wf(1));
end

== matlab function FlyingSheet_simulator/TorqueTranslator ==
  data: u_jointT input; states input; wdots input; pitchoffset input; p parameter; u_omegaL output; u_omegaR output; u_deltaL output; u_deltaR output; equivalent_gains output size=[1,3]
function [u_omegaL, u_omegaR, u_deltaL, u_deltaR, equivalent_gains] = torqueConverter(u_jointT,states, wdots, pitchoffset, p)

% The reference coming in is for angular accelleration, so don't treat it
% as pure torque:
% I*wdot = tao 

%wxr = taos(1)./p.Ix; 
%wyr = taos(2)./p.Iy;
%wzr = taos(3)./p.Iz;

tx = wdots(1)*p.Ix;
ty = wdots(2)*p.Iy;
tz = wdots(3)*p.Iz;
v = states(1:3);
vx = v(1);
vy = v(2);
vz = v(3);

omegaL = states(13);
omegaR = states(14);

%init outputs
u_deltaL = 0;
u_deltaR = 0;
u_omegaL = 0;
u_omegaR = 0;


% We assume propellers always spin one way. Never reverse.
% We know wanted torque, i.e. we know wdot*Iz=taoz=p.yt*(TL-TR)=p.yt*dT
% taoz./p.yt = TL-TR = p.K_T*(omegaL^2-omegaR^2)
% taoz/(p.yt*p.K_T) = omegaL^2-omegaR^2
% we also know
%TL = JT+dT/2
%TR = JT-dt/2
% => TL-TR = dT = taoz
% if TL=p.K_T*omegaL^2 then
%omegaL=sqrt(TL/p.K_T) =>
%omegaL=sqrt( (JT+dt/2)/p.K_T )
u_omegaL2 = (u_jointT+(tz/p.yt)/2)/p.K_T ; % THese share the jointT, half each.
u_omegaR2 =  (u_jointT-(tz/p.yt)/2)/p.K_T ;
if u_omegaL2 < 0
    u_omegaL = 0;
else
    u_omegaL = sqrt(u_omegaL2);
end
if u_omegaR2 < 0
    u_omegaR = 0;
else
    u_omegaR = sqrt(u_omegaR2);
end

% Lets make a few (crude) approximations.
% - Damping due to rotational speed doesn't exist.
% - Winglets have no z-offset.
% - Wings provide no pitch moment from lift
% Then we come to these formulas for torque around each axis:
%f1 = p.yf.*(FLT+FL -FRT-FR)
%f2 = p.xf.*(FLT+FL+FRT+FR) ...
%f3 = p.yt.*(TL-TR) ...
% 
% They essentially say that aileroins are effective proportioanlly to the
% (square) of the air velocity over them.
% Lets invert that and use as our tunable gain.

% airflow in thrust wake
v_w_L = p.b_w .* omegaL; %[b_w .* omegaL; vy; vz];
v_w_R = p.b_w .* omegaR;
% AILERONS
% Lift inside wake, signs bc rotation dir of aileron
%dFT = -p.CLdelta * 0.5*p.rho * p.Saw;% * deltaL*v_w_L.^2;
 dFT = -p.CLdelta * 0.5*p.rho * p.Saw;% * deltaR*v_w_R.^2;
% Lift outside wake
dF = -sign(vx).*p.CLdelta * 0.5*p.rho*(vx.^2 + vy.^2 + vz.^2) * p.Sa;% * deltaL;

%taoy = p.xf.*(FLT+FL+FRT+FR) ...
%taoy/p.xf = FLT+FL+FRT+FR
%taoy/p.xf = dFT*deltaL*v_w_L.^2 + dFT*deltaR*v_w_R.^2 +dF*(deltaL+deltaR);
%taoy/p.xf = dFT*jointA*v_w_L.^2 + dFT*jointA*v_w_R.^2 +dF*(2*jointA);
%taoy/p.xf = jointA(dFT*v_w_L.^2 + dFT*v_w_R.^2 +dF*2);
%taoy/(p.xf*(dFT*v_w_L.^2 + dFT*v_w_R.^2 +dF*2)) = jointA;
%%%u_jointA = ty/(p.xf*(dFT*v_w_L.^2 + dFT*v_w_R.^2 +dF*2));


%taox/p.yf = (dFLT+dFL)*deltaL - (dFRT+dFR)*deltaR;
%taox/p.yf = dF(deltaL-deltaR) + dFLT*deltaL -dFRT*deltaR;
%toax/p.yf = dF(deltaL-deltaR) + dFT*(deltaL*v_w_L.^2 - deltaR*v_w_R.^2)
%toax/p.yf = -dF*dA + dFT*(deltaL*v_w_L.^2 - deltaR*v_w_R.^2)

%deltaL = JA - dA/2; % Probably bad assumption, jump to other assumptiom
%deltaR = JA + dA/2; => 
%toax/p.yf = -dF*dA + dFT*((JA-dA/2)*v_w_L.^2 - (JA+dA/2)*v_w_R.^2)
%toax/p.yf = -dF*dA + dFT*( JA*v_w_L.^2 - dA*v_w_L.^2/2 - JA*v_w_R.^2 + dA*v_w_R.^2/2)
%toax/p.yf = -dF*dA + dFT*JA(v_w_L.^2-v_w_R.^2) - ( dA*v_w_L.^2/2  - dA*v_w_R.^2/2)
%toax/p.yf - dFT*JA(v_w_L.^2-v_w_R.^2) = -dF*dA - dA*(v_w_L.^2 -v_w_R.^2)/2
%toax/p.yf - dFT*JA(v_w_L.^2-v_w_R.^2) = -dA(dF + (v_w_L.^2 -v_w_R.^2)/2)
%-(toax/p.yf - dFT*JA(v_w_L.^2-v_w_R.^2)) / (dF + (v_w_L.^2 -v_w_R.^2)/2) = dA
%u_deltaA = -(tx/p.yf - dFT*u_jointA*(v_w_L.^2-v_w_R.^2)) / (dF + (v_w_L.^2 -v_w_R.^2)/2);

%taox/p.yf = (dFLT+dFL)*deltaL - (dFRT+dFR)*deltaR;
%taox/p.yf = dF(deltaL-deltaR) + dFLT*deltaL -dFRT*deltaR;
%toax/p.yf = dF(deltaL-deltaR) + dFT*(deltaL*v_w_L.^2 - deltaR*v_w_R.^2)
%toax/p.yf = -dF*dA + dFT*(deltaL*v_w_L.^2 - deltaR*v_w_R.^2)

%deltaL = -dA/2; % Maube correct assumption?
%deltaR = +dA/2; => 
%toax/p.yf = -dF*dA + dFT*((-dA/2)*v_w_L.^2 - (+dA/2)*v_w_R.^2)
%toax/p.yf = -dF*dA + dFT*( - dA*v_w_L.^2/2   dA*v_w_R.^2/2)
%toax/p.yf = -dF*dA - ( dA*v_w_L.^2/2  - dA*v_w_R.^2/2)
%toax/p.yf = -dF*dA - dA*(v_w_L.^2 -v_w_R.^2)/2
%toax/p.yf = -dA(dF + (v_w_L.^2 -v_w_R.^2)/2)
%-(toax/p.yf) / (dF + (v_w_L.^2 -v_w_R.^2)/2) = dA
%%%u_deltaA = -(tx/p.yf) / (dF + 0*0.5*(v_w_L.^2 -v_w_R.^2));


%u_deltaA = (365.0*(3.66e97*omegaL^2*tx + 3.66e97*omegaR^2*tx - 6.17e97*omegaL^2*ty + 6.17e97*omegaR^2*ty - 1.32e91*omegaL^3*abs(omegaL) + 1.32e91*omegaR^3*abs(omegaR) - 2.53e94*omegaL^2*vx*(vx^2 + vz^2)^(1/2) + 2.53e94*omegaR^2*vx*(vx^2 + vz^2)^(1/2) - 2.59e95*omegaL^2*vz*(vx^2 + vz^2)^(1/2) + 2.59e95*omegaR^2*vz*(vx^2 + vz^2)^(1/2) + 1.32e91*omegaL*omegaR^2*abs(omegaL) - 1.32e91*omegaL^2*omegaR*abs(omegaR) + 6.36e100*tx*vx^2*sign(vx) + 6.36e100*tx*vy^2*sign(vx) + 6.36e100*tx*vz^2*sign(vx) + 2.53e95*omegaL^2*vz*cos(2.0*atan2(1.0*vz, vx))*(vx^2 + vz^2)^(1/2) - 2.53e95*omegaR^2*vz*cos(2.0*atan2(1.0*vz, vx))*(vx^2 + vz^2)^(1/2) - 1.52e95*omegaL^2*vx*sin(2.0*atan2(1.0*vz, vx))*(vx^2 + vz^2)^(1/2) + 1.52e95*omegaR^2*vx*sin(2.0*atan2(1.0*vz, vx))*(vx^2 + vz^2)^(1/2)))/(8.21e100*vx^4*sign(vx)^2 + 8.21e100*vy^4*sign(vx)^2 + 8.21e100*vz^4*sign(vx)^2 + 1.09e95*omegaL^2*omegaR^2 + 1.64e101*vx^2*vy^2*sign(vx)^2 + 1.64e101*vx^2*vz^2*sign(vx)^2 + 1.64e101*vy^2*vz^2*sign(vx)^2 + 9.45e97*omegaL^2*vx^2*sign(vx) + 9.45e97*omegaR^2*vx^2*sign(vx) + 9.45e97*omegaL^2*vy^2*sign(vx) + 9.45e97*omegaR^2*vy^2*sign(vx) + 9.45e97*omegaL^2*vz^2*sign(vx) + 9.45e97*omegaR^2*vz^2*sign(vx));
%u_jointA = -(1.46*(4.58e99*omegaR^2*tx - 4.58e99*omegaL^2*tx + 7.71e99*omegaL^2*ty + 7.71e99*omegaR^2*ty + 1.64e93*omegaL^3*abs(omegaL) + 1.64e93*omegaR^3*abs(omegaR) + 3.16e96*omegaL^2*vx*(vx^2 + vz^2)^(1/2) + 3.16e96*omegaR^2*vx*(vx^2 + vz^2)^(1/2) + 3.24e97*omegaL^2*vz*(vx^2 + vz^2)^(1/2) + 3.24e97*omegaR^2*vz*(vx^2 + vz^2)^(1/2) + 1.64e93*omegaL*omegaR^2*abs(omegaL) + 1.64e93*omegaL^2*omegaR*abs(omegaR) + 5.49e99*vx^3*sign(vx)*(vx^2 + vz^2)^(1/2) + 5.63e100*vz^3*sign(vx)*(vx^2 + vz^2)^(1/2) + 1.34e103*ty*vx^2*sign(vx) + 1.34e103*ty*vy^2*sign(vx) + 1.34e103*ty*vz^2*sign(vx) + 5.49e99*vx*vy^2*sign(vx)*(vx^2 + vz^2)^(1/2) + 5.49e99*vx*vz^2*sign(vx)*(vx^2 + vz^2)^(1/2) + 5.63e100*vx^2*vz*sign(vx)*(vx^2 + vz^2)^(1/2) + 5.63e100*vy^2*vz*sign(vx)*(vx^2 + vz^2)^(1/2) + 2.86e96*omegaL*vx^2*abs(omegaL)*sign(vx) + 2.86e96*omegaR*vx^2*abs(omegaR)*sign(vx) + 2.86e96*omegaL*vy^2*abs(omegaL)*sign(vx) + 2.86e96*omegaR*vy^2*abs(omegaR)*sign(vx) + 2.86e96*omegaL*vz^2*abs(omegaL)*sign(vx) + 2.86e96*omegaR*vz^2*abs(omegaR)*sign(vx) - 3.16e97*omegaL^2*vz*cos(2.0*atan2(1.0*vz, vx))*(vx^2 + vz^2)^(1/2) - 3.16e97*omegaR^2*vz*cos(2.0*atan2(1.0*vz, vx))*(vx^2 + vz^2)^(1/2) + 1.9e97*omegaL^2*vx*sin(2.0*atan2(1.0*vz, vx))*(vx^2 + vz^2)^(1/2) + 1.9e97*omegaR^2*vx*sin(2.0*atan2(1.0*vz, vx))*(vx^2 + vz^2)^(1/2) - 5.49e100*vz^3*cos(2.0*atan2(1.0*vz, vx))*sign(vx)*(vx^2 + vz^2)^(1/2) + 3.29e100*vx^3*sin(2.0*atan2(1.0*vz, vx))*sign(vx)*(vx^2 + vz^2)^(1/2) - 5.49e100*vx^2*vz*cos(2.0*atan2(1.0*vz, vx))*sign(vx)*(vx^2 + vz^2)^(1/2) - 5.49e100*vy^2*vz*cos(2.0*atan2(1.0*vz, vx))*sign(vx)*(vx^2 + vz^2)^(1/2) + 3.29e100*vx*vy^2*sin(2.0*atan2(1.0*vz, vx))*sign(vx)*(vx^2 + vz^2)^(1/2) + 3.29e100*vx*vz^2*sin(2.0*atan2(1.0*vz, vx))*sign(vx)*(vx^2 + vz^2)^(1/2)))/(8.21e100*vx^4*sign(vx)^2 + 8.21e100*vy^4*sign(vx)^2 + 8.21e100*vz^4*sign(vx)^2 + 1.09e95*omegaL^2*omegaR^2 + 1.64e101*vx^2*vy^2*sign(vx)^2 + 1.64e101*vx^2*vz^2*sign(vx)^2 + 1.64e101*vy^2*vz^2*sign(vx)^2 + 9.45e97*omegaL^2*vx^2*sign(vx) + 9.45e97*omegaR^2*vx^2*sign(vx) + 9.45e97*omegaL^2*vy^2*sign(vx) + 9.45e97*omegaR^2*vy^2*sign(vx) + 9.45e97*omegaL^2*vz^2*sign(vx) + 9.45e97*omegaR^2*vz^2*sign(vx));


%u_deltaL = u_jointA - u_deltaA/2;
%u_deltaR = u_jointA + u_deltaA/2;

% Below includes pitch down moment from lift
%u_deltaL = -(1.0*(0.5*ty - 0.00102*(vx^2 + vz^2)^(1/2)*(vz*(2.0*cos(2.0*atan2(1.0*vz, vx)) - 2.05) - 1.0*vx*(1.2*sin(2.0*atan2(1.0*vz, vx)) + 0.2)) + 2.13e-7*omegaL*abs(omegaL)))/(0.00209*sign(vx)*(vx^2 + vy^2 + vz^2) + 2.41e-6*omegaL^2) - (0.5*tx)/(0.00353*sign(vx)*(vx^2 + vy^2 + vz^2) + 4.06e-6*omegaL^2);
%u_deltaR =  (0.5*tx)/(0.00353*sign(vx)*(vx^2 + vy^2 + vz^2) + 4.06e-6*omegaR^2) - (1.0*(0.5*ty - 0.00102*(vx^2 + vz^2)^(1/2)*(vz*(2.0*cos(2.0*atan2(1.0*vz, vx)) - 2.05) - 1.0*vx*(1.2*sin(2.0*atan2(1.0*vz, vx)) + 0.2)) + 2.13e-7*omegaR*abs(omegaR)))/(0.00209*sign(vx)*(vx^2 + vy^2 + vz^2) + 2.41e-6*omegaR^2);

% Below only includes sensitivity from airflow % The pitch offet is our
% mechanical trim on the aircraft.
v2 = (vx^2 + vy^2 + vz^2);
omegaL_f = omegaL; %omegas_filt(1);
omegaR_f = omegaR; %omegas_filt(2);
u_deltaL = -(0.5*ty) / (0.00209*sign(vx)*v2 + 2.41e-6*omegaL_f.^2) - (0.5*tx) / (0.00353*sign(vx)*v2 + 4.06e-6*omegaL_f.^2) + pitchoffset;
u_deltaR =  (0.5*tx) / (0.00353*sign(vx)*v2 + 4.06e-6*omegaR_f.^2) - (0.5*ty) / (0.00209*sign(vx)*v2 + 2.41e-6*omegaR_f.^2) + pitchoffset;
 

% The equivalent gains are very misleading, so don't use them much.
equivalent_gains = [ (u_deltaL-u_deltaR)./tx, 0.5*(u_deltaL+u_deltaR)./ty, ...
    (u_omegaL-u_omegaR)./tz];

== matlab function FlyingSheet_simulator/MATLAB Function5 ==
  data: angErr input; taos output; w input; hovermode input
function taos = fcn(angErr, w, hovermode)

taos = [0;0;0];

P1_fly = 4;
P2_fly = 1.5;
cx_fly = -1;
cy_fly = 1;
cz_fly = -30;

P1_hover = 4;
P2_hover = 2.5-0.5;
cx_hover = -0.6/20;
cy_hover =  0.6;
cz_hover = -120;

if hovermode
    % Emil Fresk P2 controller
    taos = -P1_hover.*angErr - P2_hover.*w;
    % Adjustment for actuators
    taos(1) = cx_hover*taos(1);
    taos(2) = cy_hover*taos(2);
    taos(3) = cz_hover*taos(3);
else
    taos = -P1_fly.*angErr - P2_fly.*w;
    taos(1) = cx_fly*taos(1);
    taos(2) = cy_fly*taos(2);
    taos(3) = cz_fly*taos(3);
end
